simulink model "przyklad1"  (R2018a)
settings: Solver=VariableStepAuto  StartTime=0.0  StopTime=10.0  RelTol=1e-3
values from neighbouring files (symbols this model uses):
  A = [0 1;-1 -2]    [przyklad1_parametry.m]    (also in zad2.m = [0.99  0.095)
  Bm = [1 0;0 1]    [przyklad1_parametry.m]
  Cm = [1 0;0 1]    [przyklad1_parametry.m]
undefined symbols (not defined in the file or in its folder): Discrete, Time
libraries: ctrlSharedLib x1
settings Model: Creator=Dominik  LastModifiedBy=Dominik

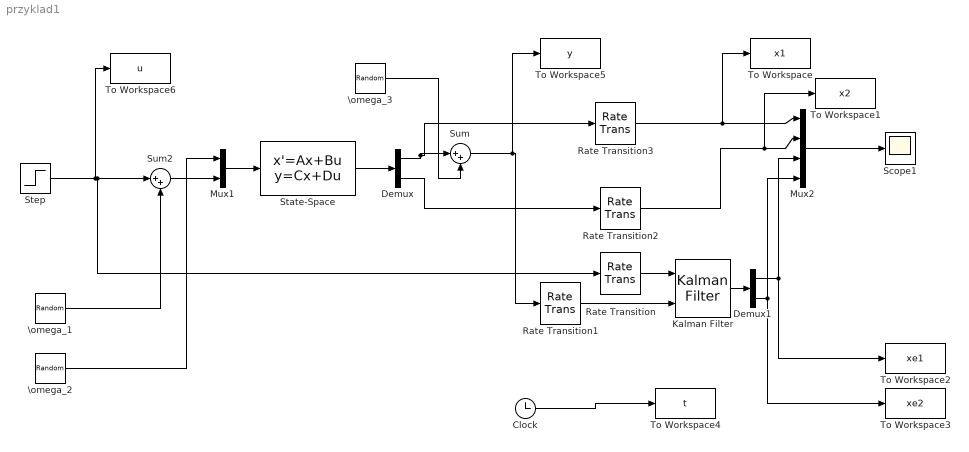
== system przyklad1 ==
  Clock : Clock
  Demux : Demux  Outputs=2
  Demux1 : Demux  Outputs=2
  Kalman Filter : ctrlSharedLib/Kalman Filter  TimeDomain=Discrete-Time  UseCurrentEstimator=on  ModelSource=LTI State-Space Variable  ModelSourceVariable=sysd  A=0.95*eye(2)  B=eye(2)  C=eye(2)  D=zeros(2)  NumberOfStates=2  NumberOfInputs=2  NumberOfOutputs=2  InitialEstimateSource=Dialog  X0=[0 0]'  P0=10*eye(2,2)  UseK=off  UseGH=off  NumberOfProcessNoiseInputs=2  G=1  TimeInvariantG=on  H=0  TimeInvariantH=on  Q=0.001*eye(2,2)  TimeInvariantQ=on  R=0.005  TimeInvariantR=on  N=0  TimeInvariantN=on  AddInputPort=on  AddEnablePort=off  OutputEstimatedY=off  OutputP=off  Ts=-1
      settings: SourceProductBaseCode=CT
  Mux1 : Mux  Inputs=2
  Mux2 : Mux
  Rate Transition{,1..3} (4 alike) : RateTransition
  Scope1 : Scope
  State-Space : StateSpace  A=A  B=Bm  C=Cm  D=zeros(2,2)  InitialCondition=[0;0]
  Step : Step  SampleTime=0
  Sum : Sum  Inputs=|++
  Sum2 : Sum  Inputs=|++
  To Workspace : ToWorkspace  VariableName=x1  SampleTime=-1
  To Workspace1 : ToWorkspace  VariableName=x2  SampleTime=-1
  To Workspace2 : ToWorkspace  VariableName=xe1  SampleTime=-1
  To Workspace3 : ToWorkspace  VariableName=xe2  SampleTime=-1
  To Workspace4 : ToWorkspace  VariableName=t  SampleTime=-1
  To Workspace5 : ToWorkspace  VariableName=y  SampleTime=-1
  To Workspace6 : ToWorkspace  VariableName=u  SampleTime=-1
  \omega_1 : RandomNumber  Variance=0.001  SampleTime=0.1
  \omega_2 : RandomNumber  Variance=0.001  Seed=23  SampleTime=0.1
  \omega_3 : RandomNumber  Variance=0.005  Seed=43  SampleTime=0.1
  wires:
  Step/1 -> Sum2/1, Rate Transition/1, To Workspace6/1
  Demux/2 -> Rate Transition2/1
  Demux/1 -> Rate Transition3/1, Sum/1
  \omega_3/1 -> Sum/2
  Kalman Filter/1 -> Demux1/1
  Mux1/1 -> State-Space/1
  Sum2/1 -> Mux1/2
  \omega_1/1 -> Sum2/2
  \omega_2/1 -> Mux1/1
  State-Space/1 -> Demux/1
  Sum/1 -> To Workspace5/1, Rate Transition1/1
  Rate Transition/1 -> Kalman Filter/1
  Rate Transition1/1 -> Kalman Filter/2
  Rate Transition3/1 -> To Workspace/1, Mux2/1
  Rate Transition2/1 -> To Workspace1/1, Mux2/2
  Mux2/1 -> Scope1/1
  Demux1/1 -> To Workspace2/1, Mux2/3
  Demux1/2 -> To Workspace3/1, Mux2/4
  Clock/1 -> To Workspace4/1
